simulink model "task1"  (R2024a)
settings: Solver=VariableStepAuto  StartTime=0.0  StopTime=10.0  RelTol=1e-3
undefined symbols (not defined in the file): T1
libraries: cstblocks x2
settings Model: Creator=lalayants  LastModifiedBy=lalayants

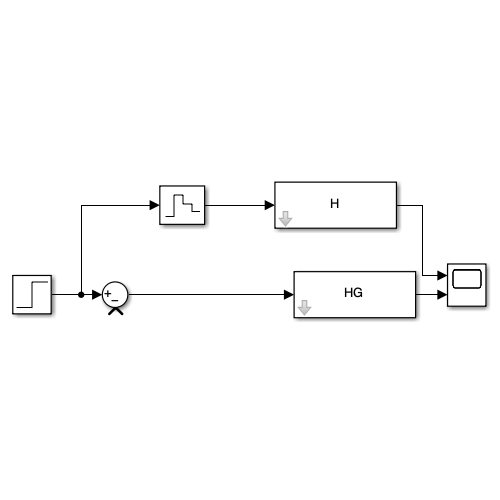
[thumbnail: Simulink's stored preview of the top-level diagram]
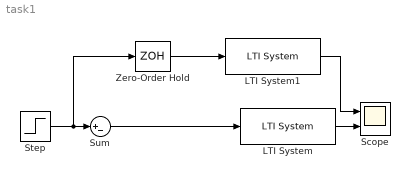
== system task1 ==
  LTI System : cstblocks/LTI System  sys=HG  IC=[]  PadeOrder=0
  LTI System1 : cstblocks/LTI System  sys=H  IC=[]  PadeOrder=0
  Scope : Scope  NumInputPorts=2
  Step : Step  Time=0  SampleTime=0
  Sum : Sum  Inputs=|+-
  Zero-Order Hold : ZeroOrderHold  SampleTime=T1
  wires:
  Step/1 -> Zero-Order Hold/1, Sum/1
  LTI System/1 -> Scope/2
  Zero-Order Hold/1 -> LTI System1/1
  LTI System1/1 -> Scope/1
  Sum/1 -> LTI System/1
